simulink model "simulation_R2018a"  (R2018a)
settings: Solver=ode1  StartTime=0.0  StopTime=3.0  FixedStep=0.001  RelTol=1e-3
values from neighbouring files (symbols this model uses):
  gamma = 2    [main.m]
  tau = 5    [main.m]
undefined symbols (not defined in the file or in its folder): sigbuilder_block
settings Model: Creator=mi4r  LastModifiedBy=tWX1242795
settings DataIOCC: ReturnWorkspaceOutputs=on
settings SFSimCC: SimUseLocalCustomCode=on
settings RTWCC: RTWUseLocalCustomCode=on

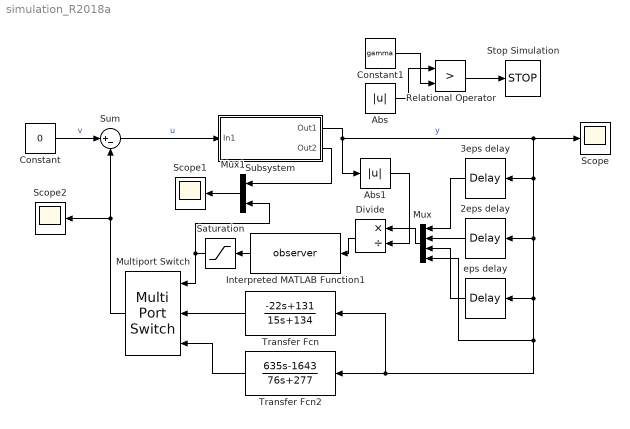
== system simulation_R2018a ==
  " eps delay" : TransportDelay  DelayTime=eps
  2eps delay : TransportDelay  DelayTime=2*eps
  3eps delay : TransportDelay  DelayTime=3*eps
  Abs : Abs
  Abs1 : Abs
  Constant : Constant  Value=0
  Constant1 : Constant  Value=gamma
  Divide : Product  Inputs=*/
  Interpreted MATLAB Function1 : MATLABFcn  MATLABFcn=observer  OutputDimensions=1
  Multiport Switch : MultiPortSwitch  Inputs=2
  Mux : Mux
  Mux1 : Mux  Inputs=2
  Relational Operator : RelationalOperator  Operator=>  OutDataTypeStr=boolean  RndMeth=Simplest
  Saturation : Saturate  UpperLimit=2  LowerLimit=1
  Scope : Scope
  Scope1 : Scope
  Scope2 : Scope
  Stop Simulation : Stop
  Subsystem : Subsystem
  Sum : Sum  Inputs=|+-
  Transfer Fcn : TransferFcn  Numerator=[-22 131]  Denominator=[15 134]
  Transfer Fcn2 : TransferFcn  Numerator=[635 -1643]  Denominator=[76 277]
  wires:
  Sum/1 -> Subsystem/1(In1)  "u"
  Constant/1 -> Sum/1  "v"
  Subsystem/1(Out1) -> Abs1/1, " eps delay"/1, Transfer Fcn/1, Transfer Fcn2/1, Mux/4, 2eps delay/1, 3eps delay/1, Scope/1  "y"
  Multiport Switch/1 -> Scope2/1, Sum/2
  Transfer Fcn/1 -> Multiport Switch/2
  Transfer Fcn2/1 -> Multiport Switch/3
  3eps delay/1 -> Mux/1
  2eps delay/1 -> Mux/2
  " eps delay"/1 -> Mux/3
  Subsystem/2(Out2) -> Mux1/1
  Mux1/1 -> Scope1/1
  Interpreted MATLAB Function1/1 -> Saturation/1
  Saturation/1 -> Multiport Switch/1, Mux1/2
  Relational Operator/1 -> Stop Simulation/1
  Constant1/1 -> Relational Operator/2
  Abs/1 -> Relational Operator/1
  Mux/1 -> Divide/1
  Abs1/1 -> Divide/2
  Divide/1 -> Interpreted MATLAB Function1/1

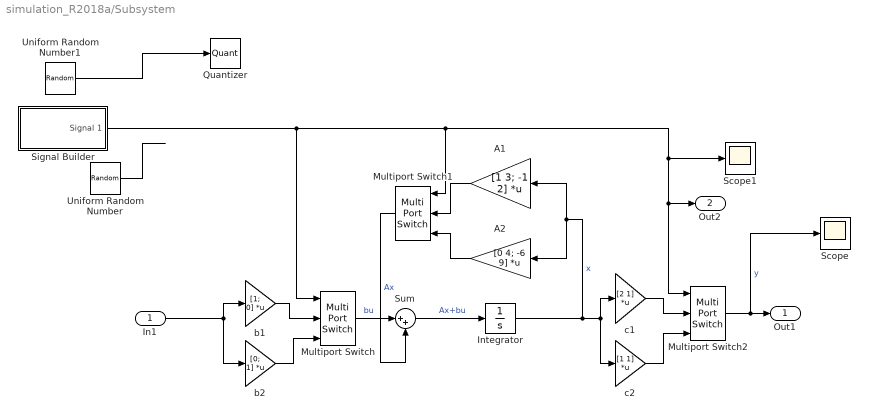
== system simulation_R2018a/Subsystem ==
  In1 : Inport
  A1 : Gain  Gain=[1 3; -1 2]  Multiplication=Matrix(K*u)
  A2 : Gain  Gain=[0 4; -6 9]  Multiplication=Matrix(K*u)
  Integrator : Integrator  InitialCondition=[0.4; 0.7]
  Multiport Switch : MultiPortSwitch  Inputs=2
  Multiport Switch1 : MultiPortSwitch  Inputs=2
  Multiport Switch2 : MultiPortSwitch  Inputs=2
  Quantizer : Quantizer  QuantizationInterval=1
  Scope : Scope
  Scope1 : Scope
  Signal Builder : Subsystem  Tag=STV Subsys  LoadFcn=sigbuilder_block('load');  StartFcn=sigbuilder_block('start');  StopFcn=sigbuilder_block('stop');  ClipboardFcn=sigbuilder_block('clipboard');  mask(Sigbuilder block){tuvar=[0:10]}
      mask help: Simulink:masks:SigbuilderBlock_MD
      mask init:
      | if ~strcmp(get_param(bdroot(gcbh),'SimulationStatus'),'stopped') tuvar = sigbuilder_block('maskInit'); end
      settings: CopyFcn=sigbuilder_block('copy');  DeleteFcn=sigbuilder_block('delete');  ModelCloseFcn=sigbuilder_block('modelClose');  PreSaveFcn=sigbuilder_block('preSave');  PauseFcn=sigbuilder_block('pause');  ContinueFcn=sigbuilder_block('continue');  NameChangeFcn=sigbuilder_block('namechange');  OpenFcn=sigbuilder_block('open',[396.6 99.6 550.8 400.2 ]);  CloseFcn=sigbuilder_block('close');
      mask Display: plot(0, 0, 100, 100,[2, 2, 32, 32, 2], [68, 8, 8, 68, 68],[32, 2], [38, 38], [32, 19, 2],[53, 60, 44], [32, 17, 17, 2],[16, 16, 31, 31]);txt = getActiveGroup(gcbh);text(2, 100, txt,'verticalAlignment', 'top');
  Sum : Sum  Inputs=|++
  Uniform Random Number : UniformRandomNumber  Minimum=tau  Maximum=10*tau  SampleTime=0.1
  Uniform Random Number1 : UniformRandomNumber  Minimum=1  Maximum=2  SampleTime=0.1
  b1 : Gain  Gain=[1; 0]  Multiplication=Matrix(K*u)
  b2 : Gain  Gain=[0; 1]  Multiplication=Matrix(K*u)
  c1 : Gain  Gain=[2 1]  Multiplication=Matrix(K*u)
  c2 : Gain  Gain=[1 1]  Multiplication=Matrix(K*u)
  Out1 : Outport
  Out2 : Outport  Port=2
  wires:
  In1/1 -> b2/1, b1/1
  Multiport Switch/1 -> Sum/1  "bu"
  Sum/1 -> Integrator/1  "Ax+bu"
  Integrator/1 -> c2/1, c1/1, A2/1, A1/1  "x"
  c1/1 -> Multiport Switch2/2
  c2/1 -> Multiport Switch2/3
  Multiport Switch2/1 -> Scope/1, Out1/1  "y"
  b2/1 -> Multiport Switch/3
  b1/1 -> Multiport Switch/2
  A1/1 -> Multiport Switch1/2
  A2/1 -> Multiport Switch1/3
  Multiport Switch1/1 -> Sum/2  "Ax"
  Signal Builder/1(Signal 1) -> Multiport Switch/1, Multiport Switch1/1, Out2/1, Multiport Switch2/1, Scope1/1
  Uniform Random Number/1 -> ?
  Uniform Random Number1/1 -> Quantizer/1

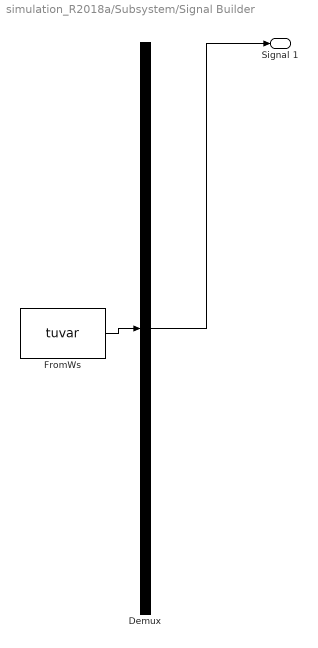
== system simulation_R2018a/Subsystem/Signal Builder ==
  Demux : Demux  Tag=STV Demux  Outputs=1
      settings: DisplayOption=none
  FromWs : FromWorkspace  Tag=STV FromWs  VariableName=tuvar
      SigBuilderData=|
      | common.afterFinalStr = 'Extrapolate'
      | common.sampleTime = 0
      | dataSet.timeRange = [0 10]
      | dataSet.name = 'Group 1'
      | sbobj.Groups.Name = 'Group 1'
      | sbobj.Groups.Signals.Name = 'Signal 1'
      | sbobj.Groups.Signals.XData = [0 0.8 0.8 1.96 1.96 10]
      | sbobj.Groups.Signals.YData = [1 1 2 2 1 1]
  Signal 1 : Outport  Tag=STV Outport
  wires:
  Demux/1 -> Signal 1/1
  FromWs/1 -> Demux/1
